simulink model "Exp8"  (R2018a)
settings: Solver=VariableStepAuto  StartTime=0.0  StopTime=1  RelTol=1e-3
libraries: powerlib x6, powerlib_meascontrol x6
settings Model: Creator=Asus  LastModifiedBy=Asus

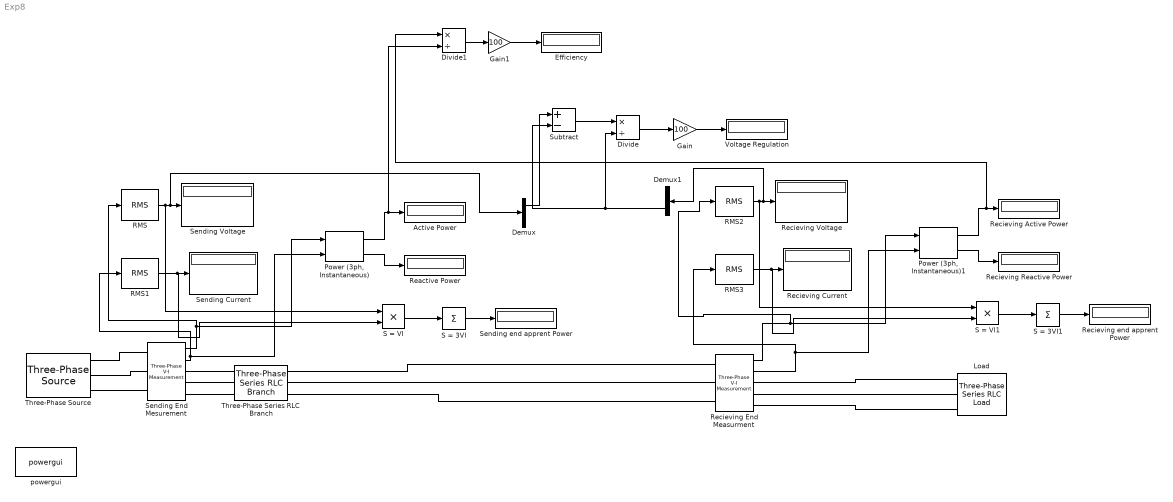
== system Exp8 ==
  Active Power : Display
  Demux : Demux  Outputs=3
  Demux1 : Demux  Outputs=3
  Divide : Product  Inputs=*/
  Divide1 : Product  Inputs=*/
  "Efficiency " : Display
  Gain : Gain  Gain=100
  Gain1 : Gain  Gain=100
  Load : powerlib/Elements/Three-Phase Series RLC Load  LConnTagsString=A|B|C  Configuration=Y (grounded)  NominalVoltage=220e3  Vabc=[1e3 1e3 1e3]  Vabcp=[1e3 1e3 1e3]  NominalFrequency=60  UnbalancedPower=off  ActivePower=304.8e6  InductivePower=228.6e6  CapacitivePower=0  Pabc=[10e3 9e3 11e3]  QLabc=[100 90 110]  QCabc=[100 90 110]  Pabcp=[10e3 9e3 11e3]  QLabcp=[100 90 110]  QCabcp=[100 90 110]  Measurements=None  LoadType=constant Z
  "Power (3ph, Instantaneous)" : powerlib_meascontrol/Measurements/Power (3ph, Instantaneous)
      settings: SourceProductName=Simscape Power Systems
  "Power (3ph, Instantaneous)1" : powerlib_meascontrol/Measurements/Power (3ph, Instantaneous)
      settings: SourceProductName=Simscape Power Systems
  RMS{,1..3} (4 alike) : powerlib_meascontrol/Measurements/RMS  TrueRMS=on  Freq=60  RMSInit=0  Ts=0
  Reactive Power : Display
  Recieving Reactive Power : Display
  Recieving Active Power : Display
  "Recieving Current " : Display
  Recieving End Measurment : powerlib/Measurements/Three-Phase V-I Measurement  VoltageMeasurement=phase-to-ground  SetLabelV=off  LabelV=Vabc  Vpu=off  VpuLL=off  CurrentMeasurement=yes  SetLabelI=off  LabelI=Iabc  Ipu=off  Pbase=100e6  Vbase=500e3  OutputType=Complex  PhasorSimulation=off  PSBequivalent=0
  "Recieving Voltage " : Display
  Recieving end apprent Power : Display
  S = 3VI : Sum  Inputs=+
  S = 3VI1 : Sum  Inputs=+
  S = VI : Product
  S = VI1 : Product
  "Sending Current " : Display
  Sending End Mesurement : powerlib/Measurements/Three-Phase V-I Measurement  VoltageMeasurement=phase-to-ground  SetLabelV=off  LabelV=Vabc  Vpu=off  VpuLL=off  CurrentMeasurement=yes  SetLabelI=off  LabelI=Iabc  Ipu=off  Pbase=100e6  Vbase=500e3  OutputType=Complex  PhasorSimulation=off  PSBequivalent=0
  "Sending Voltage " : Display
  Sending end apprent Power : Display
  Subtract : Sum  Inputs=+-
  Three-Phase Series RLC Branch : powerlib/Elements/Three-Phase Series RLC Branch  LConnTagsString=A|B|C  RConnTagsString=A|B|C  BranchType=RL  Resistance=6  Inductance=0.053052  Capacitance=1e-6  Measurements=None
  Three-Phase Source : powerlib/Electrical Sources/Three-Phase Source  InternalConnection=Yg  VoltagePhases=off  Voltage=250e3  PhaseAngle=0  Voltage_phases=[25e3 25e3 25e3]/sqrt(3)  PhaseAngles_phases=[0 -120 +120]  Frequency=60  NonIdealSource=off  SpecifyImpedance=off  Resistance=0.8929  Inductance=16.58e-3  ShortCircuitLevel=100e6  BaseVoltage=25e3  XRratio=7  BusType=swing  Pref=10e3  Qref=0  Prefabc=[10e3, 10e3, 10e3]  Qrefabc=[0, 0, 0]  Qmin=-inf  Qmax=inf
  Voltage Regulation : Display
  powergui : powerlib/powergui  Priority=1  SimulationMode=Continuous  SampleTime=50e-6  frequency=60  Iterations=50  frequencyindice=60  Pbase=100e6  ErrMax=1e-4  UnitsV=kV  UnitsW=MW  buscounter=0  FunctionMessages=off  echomessages=off  EnableUseOfTLC=off  CurrentSourceSwitches=off  DisableSnubberDevices=off  DisableRonSwitches=off  DisableVfSwitches=off  DisplayEquations=off  SolverType=Tustin/Backward Euler (TBE)  Interpol=off  ExternalGateDelay=off  methode=off  Ts=100  x0status=blocks  SPID=on  SwTol=0  HookPort=off  RestoreLinks=warning  ResistiveCurrentMeasurement=off  Frange=[0:2:500]  Ylog=off  Xlog=on  ShowGrid=off  save=off  variable=ZData  structure=0  ZoomFFT=off  StartTime=0.0  cycles=1  DisplayStyle=1  fundamental=60  FreqAxis=off  MaxFrequency=1000  frequencyindicesteady=1  RmsSteady=1  display=off
  wires:
  Sending End Mesurement/1 -> "Power (3ph, Instantaneous)"/1, RMS/1
  RMS/1 -> S = VI/1, Demux/1, "Sending Voltage "/1
  RMS1/1 -> S = VI/2, "Sending Current "/1
  Sending End Mesurement/2 -> "Power (3ph, Instantaneous)"/2, RMS1/1
  "Power (3ph, Instantaneous)"/1 -> Divide1/2, Active Power/1
  "Power (3ph, Instantaneous)"/2 -> Reactive Power/1
  S = VI/1 -> S = 3VI/1
  S = 3VI/1 -> Sending end apprent Power/1
  RMS2/1 -> S = VI1/1, Demux1/1, "Recieving Voltage "/1
  RMS3/1 -> S = VI1/2, "Recieving Current "/1
  Recieving End Measurment/1 -> "Power (3ph, Instantaneous)1"/1, RMS2/1
  "Power (3ph, Instantaneous)1"/2 -> Recieving Reactive Power/1
  "Power (3ph, Instantaneous)1"/1 -> Divide1/1, Recieving Active Power/1
  Recieving End Measurment/2 -> RMS3/1, "Power (3ph, Instantaneous)1"/2
  S = VI1/1 -> S = 3VI1/1
  S = 3VI1/1 -> Recieving end apprent Power/1
  Demux/1 -> Subtract/1
  Demux1/3 -> Divide/2, Subtract/2
  Subtract/1 -> Divide/1
  Divide/1 -> Gain/1
  Gain/1 -> Voltage Regulation/1
  Divide1/1 -> Gain1/1
  Gain1/1 -> "Efficiency "/1
  connections:
  Three-Phase Source/RConn1 -- Sending End Mesurement/LConn1
  Three-Phase Source/RConn2 -- Sending End Mesurement/LConn2
  Three-Phase Source/RConn3 -- Sending End Mesurement/LConn3
  Sending End Mesurement/RConn1 -- Three-Phase Series RLC Branch/LConn1
  Sending End Mesurement/RConn2 -- Three-Phase Series RLC Branch/LConn2
  Sending End Mesurement/RConn3 -- Three-Phase Series RLC Branch/LConn3
  Three-Phase Series RLC Branch/RConn1 -- Recieving End Measurment/LConn1
  Three-Phase Series RLC Branch/RConn2 -- Recieving End Measurment/LConn2
  Three-Phase Series RLC Branch/RConn3 -- Recieving End Measurment/LConn3
  Recieving End Measurment/RConn1 -- Load/LConn1
  Recieving End Measurment/RConn2 -- Load/LConn2
  Recieving End Measurment/RConn3 -- Load/LConn3
